simulink model "compareModels"  (R2022a)
settings: Solver=VariableStepAuto  StartTime=0.0  StopTime=168  RelTol=1e-3
model workspace (MAT data in the model file):
  Q_in = [0.12271780758; 0.123470790595; 0.124228393831; 0.124990645638; 0.125757574538; 0.12652920923; 0.127305578587]
  Sig = Simulink.Signal
  Sig.DataType = 'auto'
  Sig.Dimensions = -1
  Sig.DimensionsMode = 'auto'
  Sig.Complexity = 'auto'
  Sig.SampleTime = -1
  Sig.SamplingMode = 'auto'
  Y_mAb_X = 3.05833848775e-12
  mnt_mAb = 1.19887616406e-08
  x0 = [0.2; 200000000; 200000000; 25.1; 5.01; 0; 0; 100; 0; 0; 0; 0; 0; 0; 0; 0]
  xR0 = [0.2; 200000000; 200000000; 25.1; 5.01; 0; 0; 100]
libraries: simulink x1
settings Model: Creator=tomok  LastModifiedBy=tomok

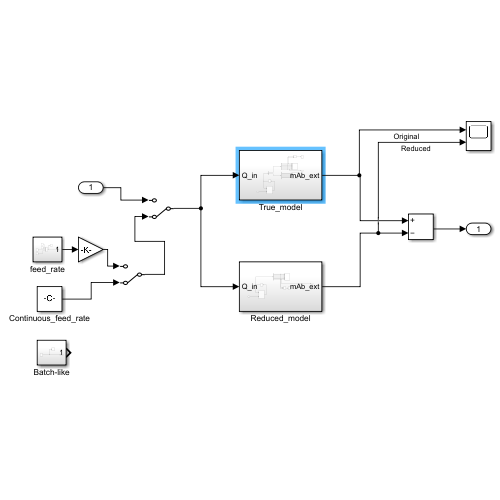
[thumbnail: Simulink's stored preview of the top-level diagram]
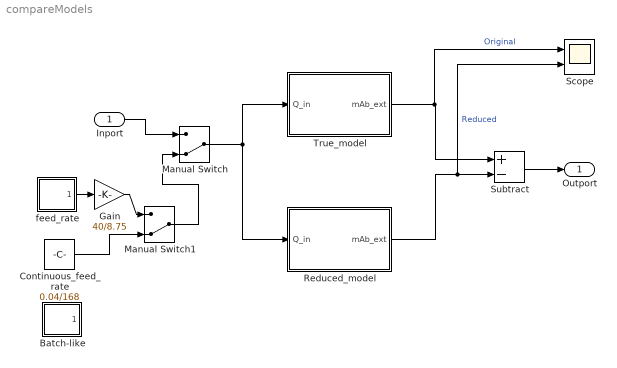
== system compareModels ==
  Inport : Inport
  Batch-like : Subsystem
  Continuous_feed_rate : Constant  Value=0.04/168
  Gain : Gain  Gain=40/8.75
  Manual Switch : ManualSwitch  CurrentSetting=0
  Manual Switch1 : ManualSwitch  CurrentSetting=0
  Reduced_model : Subsystem
  Scope : Scope  NumInputPorts=2
  Subtract : Sum  Inputs=+-
  True_model : Subsystem
  feed_rate : Subsystem
  Outport : Outport
  wires:
  True_model/1(mAb_ext) -> Scope/1, Subtract/1  "Original"
  Reduced_model/1(mAb_ext) -> Scope/2, Subtract/2  "Reduced"
  Subtract/1 -> Outport/1
  Inport/1 -> Manual Switch/1
  feed_rate/1(Out1) -> Gain/1
  Manual Switch/1 -> Reduced_model/1(Q_in), True_model/1(Q_in)
  Manual Switch1/1 -> Manual Switch/2
  Gain/1 -> Manual Switch1/1
  Continuous_feed_rate/1 -> Manual Switch1/2

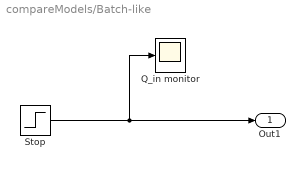
== system compareModels/Batch-like ==
  Q_in monitor : Scope
  Stop : Step  Time=0.01  Before=0.04/0.01  After=0  SampleTime=0
  Out1 : Outport
  wires:
  Stop/1 -> Q_in monitor/1, Out1/1

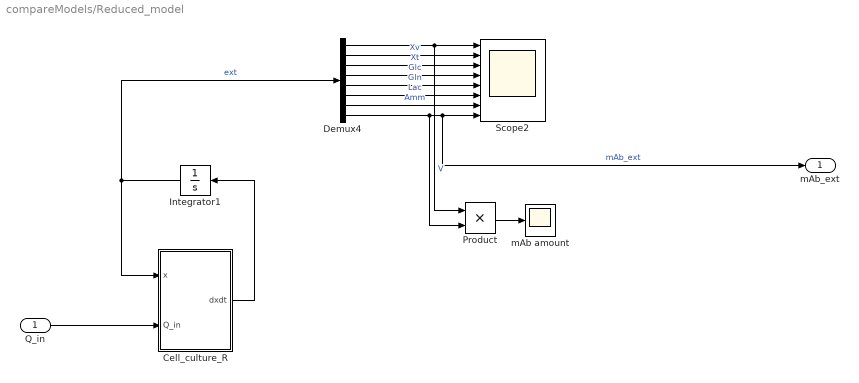
== system compareModels/Reduced_model ==
  Q_in : Inport
  Cell_culture_R : MATLAB Function  TreatAsAtomicUnit=on
  Demux4 : Demux  Outputs=8
  Integrator1 : Integrator  InitialCondition=xR0  LimitOutput=on  LowerSaturationLimit=0
  Product : Product
  Scope2 : Scope  NumInputPorts=8
  mAb amount : Scope
  mAb_ext : Outport
  wires:
  Demux4/8 -> Product/2, mAb_ext/1, Scope2/8  "mAb_ext"
  Demux4/4 -> Scope2/4  "Glc"
  Demux4/6 -> Scope2/6  "Lac"
  Demux4/7 -> Scope2/7  "Amm"
  Demux4/3 -> Scope2/3  "Xt"
  Demux4/2 -> Scope2/2  "Xv"
  Integrator1/1 -> Demux4/1, Cell_culture_R/1(x)  "ext"
  Demux4/1 -> Product/1, Scope2/1  "V"
  Cell_culture_R/1(dxdt) -> Integrator1/1
  Demux4/5 -> Scope2/5  "Gln"
  Q_in/1 -> Cell_culture_R/2(Q_in)
  Product/1 -> mAb amount/1

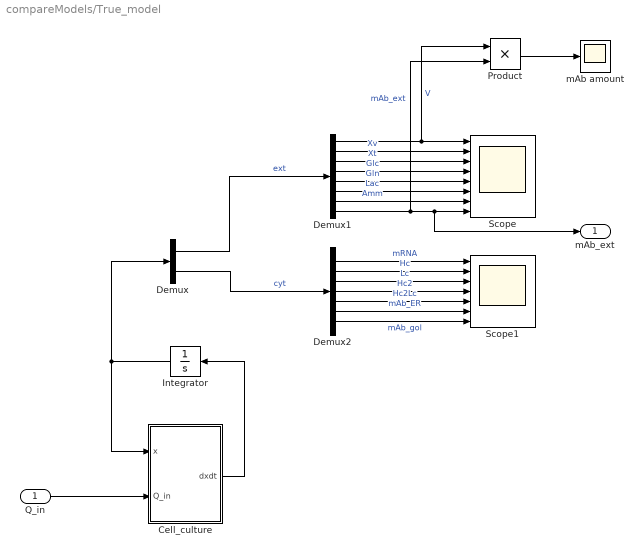
== system compareModels/True_model ==
  Q_in : Inport
  Cell_culture : MATLAB Function  TreatAsAtomicUnit=on
  Demux : Demux  Outputs=[8 8]
  Demux1 : Demux  Outputs=8
  Demux2 : Demux  Outputs=[2 1 1 1 1 1 1]
  Integrator : Integrator  InitialCondition=x0  LimitOutput=on  LowerSaturationLimit=0
  Product : Product
  Scope : Scope  NumInputPorts=8
  Scope1 : Scope  NumInputPorts=7
  mAb amount : Scope
  mAb_ext : Outport
  wires:
  Demux2/2 -> Scope1/2  "Hc"
  Demux2/1 -> Scope1/1  "mRNA"
  Demux1/2 -> Scope/2  "Xv"
  Demux1/6 -> Scope/6  "Lac"
  Integrator/1 -> Demux/1, Cell_culture/1(x)
  Demux1/3 -> Scope/3  "Xt"
  Demux1/7 -> Scope/7  "Amm"
  Demux/1 -> Demux1/1  "ext"
  Demux2/5 -> Scope1/5  "Hc2Lc"
  Demux2/7 -> Scope1/7  "mAb_gol"
  Cell_culture/1(dxdt) -> Integrator/1
  Demux2/4 -> Scope1/4  "Hc2"
  Demux1/4 -> Scope/4  "Glc"
  Demux/2 -> Demux2/1  "cyt"
  Demux2/3 -> Scope1/3  "Lc"
  Demux2/6 -> Scope1/6  "mAb_ER"
  Demux1/5 -> Scope/5  "Gln"
  Q_in/1 -> Cell_culture/2(Q_in)
  Demux1/1 -> Product/1, Scope/1  "V"
  Demux1/8 -> Product/2, mAb_ext/1, Scope/8  "mAb_ext"
  Product/1 -> mAb amount/1

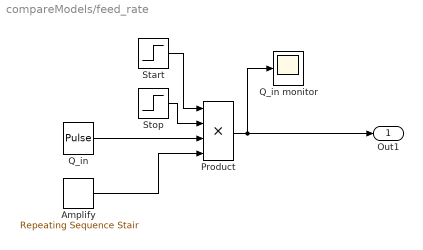
== system compareModels/feed_rate ==
  Amplify : simulink/Sources/Repeating Sequence Stair  OutValues=Q_in  tsamp=24  OutMin=[]  OutMax=[]  OutDataTypeStr=double  OutputDataTypeScalingMode=double  OutDataType=fixdt(0,8)  ConRadixGroup=Best Precision: Vector-wise  OutScaling=2^-12
  Product : Product  Inputs=4
  Q_in : DiscretePulseGenerator  PulseType=Time based  Period=24  PulseWidth=1/24  PhaseDelay=12
  Q_in monitor : Scope
  Start : Step  SampleTime=0
  Stop : Step  Time=169  Before=1  After=0  SampleTime=0
  Out1 : Outport
  wires:
  Stop/1 -> Product/2
  Start/1 -> Product/1
  Product/1 -> Q_in monitor/1, Out1/1
  Q_in/1 -> Product/3
  Amplify/1 -> Product/4

== matlab function compareModels/Reduced_model/Cell_culture_R ==
  data: dxdt output; x input; Q_in input
function dxdt = fcn(x,Q_in)
dxdt = Kontoravdi2010RStateFcn(x,Q_in);
end

== matlab function compareModels/True_model/Cell_culture ==
  data: dxdt output; x input; Q_in input
function dxdt = fcn(x,Q_in)
dxdt = Kontoravdi2010StateFcn(x,Q_in);
end
